simulink model "sim_model_ss_LQ"  (R2018b)
settings: Solver=VariableStepAuto  StartTime=0.0  StopTime=10.0  RelTol=1e-3
values from neighbouring files (symbols this model uses):
  A = J    [Main.m]
  B = [0;0;K6]    [Main.m]
  C = [1, 0, 0]    [Main.m]
  D = 0    [Main.m]
  Klq = lqr(A,B,Q,Rc)    [Main.m]
  x10 = 0.03    [Main.m]
  x20 = v0    (= 0)    [Main.m]
  x30 = I0    [Main.m]
settings Model: Creator=Eduardo  LastModifiedBy=ohara

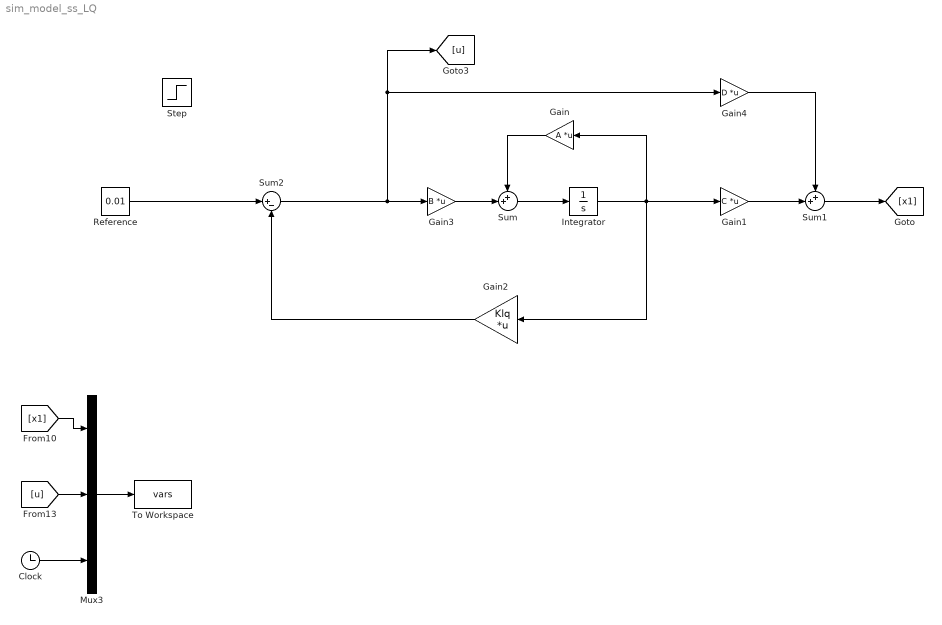
== system sim_model_ss_LQ ==
  Clock : Clock
  Gain : Gain  Gain=A  Multiplication=Matrix(K*u)
  Gain1 : Gain  Gain=C  Multiplication=Matrix(K*u)
  Gain2 : Gain  Gain=Klq  Multiplication=Matrix(K*u)
  Gain3 : Gain  Gain=B  Multiplication=Matrix(K*u)
  Gain4 : Gain  Gain=D  Multiplication=Matrix(K*u)
  Integrator : Integrator  InitialCondition=[x10;x20;x30]
  Mux3 : Mux  Inputs=3
  "Reference " : Constant  Value=0.01
  Step : Step  Time=3  SampleTime=0
  Sum : Sum  Inputs=++|
  Sum1 : Sum  Inputs=++|
  Sum2 : Sum  Inputs=|+-
  To Workspace : ToWorkspace  VariableName=vars  SaveFormat=Timeseries  SampleTime=-1
  wires:
  Sum/1 -> Integrator/1
  Gain3/1 -> Sum/2
  Gain/1 -> Sum/1
  Integrator/1 -> Gain2/1, Gain1/1, Gain/1
  Gain1/1 -> Sum1/2
  Sum1/1 -> [x1]
  [x1] -> Mux3/1
  Mux3/1 -> To Workspace/1
  [u] -> Mux3/2
  Clock/1 -> Mux3/3
  Gain2/1 -> Sum2/2
  Sum2/1 -> Gain3/1, Gain4/1, [u]
  Gain4/1 -> Sum1/1
  "Reference "/1 -> Sum2/1
